simulink library "Opto"  (R2019a)
settings: Solver=VariableStepAuto  StartTime=0.0  StopTime=10.0  RelTol=1e-3
undefined symbols (not defined in the file or in its folder): Ts
libraries: arduinolib x6, dspstat3 x2
settings Model: Creator=Gergely  LastModifiedBy=Gergely
settings DataIOCC: ReturnWorkspaceOutputs=off
settings DebuggingCC: PregeneratedLibrarySubsystemCodeDiagnostic=none  ArithmeticOperatorsInVariantConditions=warning
settings SFSimCC: SimUseLocalCustomCode=off
settings RTWCC: RTWUseLocalCustomCode=off

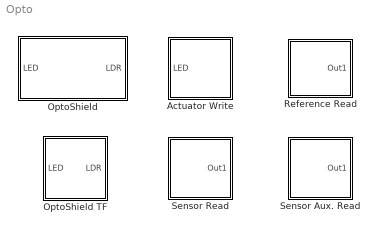
== system Opto ==
  Actuator Write : Subsystem
      mask DialogControl DescGroupVar Prompt: OptoShield LED
      mask DialogControl DescTextVar Prompt: Sets the brightness of the LEDs on the OptoShield. Expects input in the range of 0-100%.
      mask Display: image('assets\OptoShield_LED.svg');
  OptoShield : Subsystem  mask{Ts=0.01, Tcal=3}
      mask prompts: Ts "Sampling period (s):"; Tcal "Calibration time (s):"
      mask DialogControl DescGroupVar Prompt: OptoShield
      mask DialogControl DescTextVar Prompt: The block represents the OptoShield device. It accepts an input signal in the range of 0-100% and outputs a sensor reading in the range scaled to 0-100%. The block requires a sampling period and a calibration time at the beginning of the experiment allowing for the LDR to settle.
      mask Display: image('assets\OptoShield.svg');
  OptoShield TF : Subsystem
      mask DialogControl DescGroupVar Prompt: OptoShield TF
      mask DialogControl DescTextVar Prompt: The block represents the simplified first-order continuous transfer function of the OptoShield device. Both input and output are scaled to percents. The real process dynamics is nonlinear and hysteretic.
      mask Display: image('assets\OptoShield_TF.svg');
  Reference Read : Subsystem  mask{ReadoutRadio=Percentage, Ts=0.01}
      mask prompts: ReadoutRadio "Readout type"; Ts "Sample time (s):"
      mask init:
      | % Voltage
      | if ReadoutRadio==1
      | ADC_Gain=(100.0/1024);
      | end
      | 
      | % Voltage
      | if ReadoutRadio==2
      | ADC_Gain=(5.0/1024);
      | end
      | 
      | % ADC levels
      | if ReadoutRadio==3
      | ADC_Gain=1.0;
      | end
      mask TypeOptions ReadoutRadio: Percentage | Voltage | ADC levels
      mask DialogControl DescGroupVar Prompt: OptoShield Potentiometer
      mask DialogControl DescTextVar Prompt: The block represents the potentiometer on the OptoShield device. You may select the type of output scaling, depending on your needs.
      mask DialogControl Container2 Prompt: Parameters
      mask Display: image('assets\Potentiometer.svg');
  Sensor Aux. Read : Subsystem  mask{ReadoutRadio=Voltage, Ts=0.01}
      mask prompts: ReadoutRadio "Readout type"; Ts "Sample time (s):"
      mask init:
      | % Voltage
      | if ReadoutRadio==1
      | ADC_Gain=(5.0/1024);
      | end
      | 
      | % ADC levels
      | if ReadoutRadio==2
      | ADC_Gain=1.0;
      | end
      mask TypeOptions ReadoutRadio: Voltage | ADC levels
      mask DialogControl DescGroupVar Prompt: OptoShield LDR
      mask DialogControl DescTextVar Prompt: The block represents the main light-dependent resistor of the OptoShield device. You may select the type of output scaling, depending on your needs.
      mask DialogControl Container2 Prompt: Parameters
      mask Display: image('assets\OptoShield_LDR_EXT.svg');
  Sensor Read : Subsystem  mask{ReadoutRadio=Manual calibration, MaxLDR=860, Parameter3=0.01}
      mask prompts: ReadoutRadio "Readout type"; MaxLDR "Maximal LDR ADC level"; Parameter3 "Sample time (s):"
      mask init:
      | % Manual calibration
      | if ReadoutRadio==1
      | ADC_Gain=MaxLDR/100;
      | end
      | 
      | % Voltage
      | if ReadoutRadio==2
      | ADC_Gain=(5.0/1024);
      | end
      | 
      | % ADC levels
      | if ReadoutRadio==3
      | ADC_Gain=1.0;
      | end
      mask TypeOptions ReadoutRadio: Manual calibration | Voltage | ADC levels
      mask DialogControl DescGroupVar Prompt: OptoShield LDR
      mask DialogControl DescTextVar Prompt: The block represents the main light-dependent resistor of the OptoShield device. You may select the type of output scaling, depending on your needs.
      mask DialogControl Container2 Prompt: Manual calibration
      mask DialogControl Container3 Prompt: Parameters
      mask Display: image('assets\OptoShield_LDR.svg');

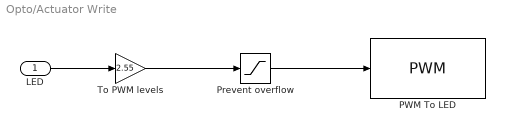
== system Opto/Actuator Write ==
  LED : Inport
  PWM To LED : arduinolib/PWM  pinNumber=3  EnableInputFrequency=off  InitialFrequency=2000  InitialDutyCycle=0  NotificationType=None  blockPlatform=arduino
  Prevent overflow : Saturate  UpperLimit=255  LowerLimit=0
  To PWM levels : Gain  Gain=2.55
  wires:
  LED/1 -> To PWM levels/1
  Prevent overflow/1 -> PWM To LED/1
  To PWM levels/1 -> Prevent overflow/1

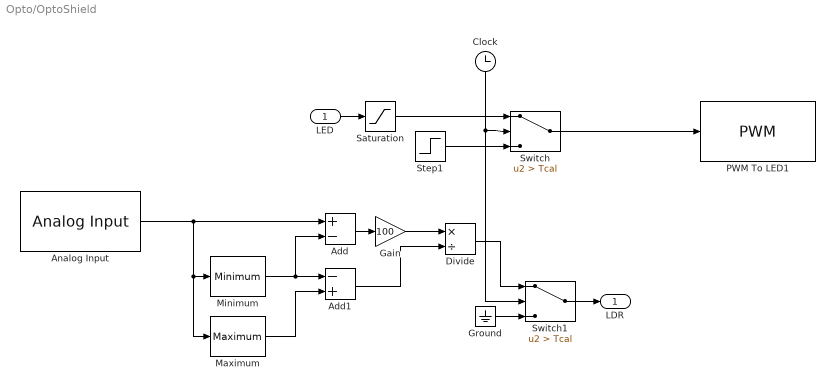
== system Opto/OptoShield ==
  LED : Inport
  Add : Sum  Inputs=+-
  Add1 : Sum  Inputs=-+
  Analog Input : arduinolib/Analog Input  pinNumber=1  ReadResultsOnly=off  ConversionTriggerSource=Software  ExternalTriggerType=uint32(0)  OutputDataType=uint16  EnableConversionCompleteNotify=off  EnableOuputStatus=off  SampleTime=Ts  blockPlatform=arduino
  Clock : Clock
  Divide : Product  Inputs=*/
  Gain : Gain  Gain=100
  Ground : Ground
  Maximum : dspstat3/Maximum  operation=maximum  fcn=Running  indexBase=One  operateOver=Each column  Dimension=1  reset=None  roiEnable=off  roiType=Rectangles  roiPortion=Entire ROI  roiOutput=Individual statistics for each ROI  roiFlag=off  roundingMode=Floor  overflowMode=off  accumDataTypeStr=Inherit: Same as product output  accumLastDataTypeStr=Inherit: Same as product output
  Minimum : dspstat3/Minimum  operation=minimum  fcn=Running  indexBase=One  operateOver=Each column  Dimension=1  reset=None  roiEnable=off  roiType=Rectangles  roiPortion=Entire ROI  roiOutput=Individual statistics for each ROI  roiFlag=off  roundingMode=Floor  overflowMode=off
      settings: SourceProductName=DSP System Toolbox  SourceProductBaseCode=DS
  PWM To LED1 : arduinolib/PWM  pinNumber=3  EnableInputFrequency=off  InitialFrequency=2000  InitialDutyCycle=0  NotificationType=None  blockPlatform=arduino
  Saturation : Saturate  UpperLimit=100  LowerLimit=0
  Step1 : Step  Time=round((0.8*Tcal/2)/Ts)*Ts  After=255  SampleTime=Ts
  Switch : Switch  Criteria=u2 > Threshold  Threshold=Tcal
  Switch1 : Switch  Criteria=u2 > Threshold  Threshold=Tcal
  LDR : Outport
  wires:
  Minimum/1 -> Add1/1, Add/2
  Maximum/1 -> Add1/2
  Clock/1 -> Switch/2, Switch1/2
  LED/1 -> Saturation/1
  Add/1 -> Gain/1
  Add1/1 -> Divide/2
  Gain/1 -> Divide/1
  Switch/1 -> PWM To LED1/1
  Analog Input/1 -> Minimum/1, Maximum/1, Add/1
  Step1/1 -> Switch/3
  Divide/1 -> Switch1/1
  Ground/1 -> Switch1/3
  Switch1/1 -> LDR/1
  Saturation/1 -> Switch/1

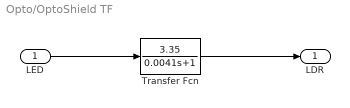
== system Opto/OptoShield TF ==
  LED : Inport
  Transfer Fcn : TransferFcn  Numerator=[3.35]  Denominator=[0.0041 1]
  LDR : Outport
  wires:
  LED/1 -> Transfer Fcn/1
  Transfer Fcn/1 -> LDR/1

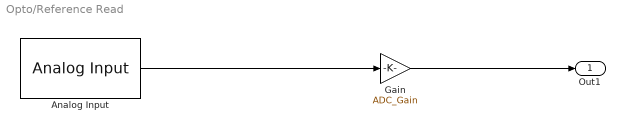
== system Opto/Reference Read ==
  Analog Input : arduinolib/Analog Input  pinNumber=0  ReadResultsOnly=off  ConversionTriggerSource=Software  ExternalTriggerType=uint32(0)  OutputDataType=uint16  EnableConversionCompleteNotify=off  EnableOuputStatus=off  SampleTime=Ts  blockPlatform=arduino
  Gain : Gain  Gain=ADC_Gain
  Out1 : Outport
  wires:
  Analog Input/1 -> Gain/1
  Gain/1 -> Out1/1

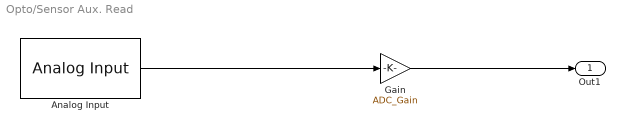
== system Opto/Sensor Aux. Read ==
  Analog Input : arduinolib/Analog Input  pinNumber=2  ReadResultsOnly=off  ConversionTriggerSource=Software  ExternalTriggerType=uint32(0)  OutputDataType=uint16  EnableConversionCompleteNotify=off  EnableOuputStatus=off  SampleTime=Ts  blockPlatform=arduino
  Gain : Gain  Gain=ADC_Gain
  Out1 : Outport
  wires:
  Analog Input/1 -> Gain/1
  Gain/1 -> Out1/1

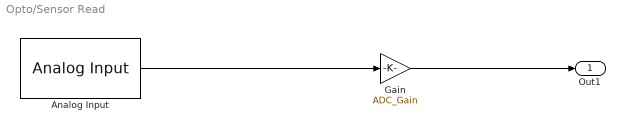
== system Opto/Sensor Read ==
  Analog Input : arduinolib/Analog Input  pinNumber=1  ReadResultsOnly=off  ConversionTriggerSource=Software  ExternalTriggerType=uint32(0)  OutputDataType=uint16  EnableConversionCompleteNotify=off  EnableOuputStatus=off  SampleTime=Ts  blockPlatform=arduino
  Gain : Gain  Gain=ADC_Gain
  Out1 : Outport
  wires:
  Analog Input/1 -> Gain/1
  Gain/1 -> Out1/1
